simulink model "TST_SmkLim_InjMassLim"  (R2016b)
settings: Solver=FixedStepDiscrete  StartTime=0.0  StopTime=4  FixedStep=sampleTime  RelTol=1e-3
values from neighbouring files (symbols this model uses):
  testCase = 1    [initTST_SmkLim_InjMassLim_001.m]    (also in initTST_SmkLim_InjMassLim_002.m = 2)
libraries: simulink x7, UnitTest_Lib x4
settings Model: Creator=zhengjinyan  LastModifiedBy=zhengjinyan
settings DebuggingCC: SignalRangeChecking=error

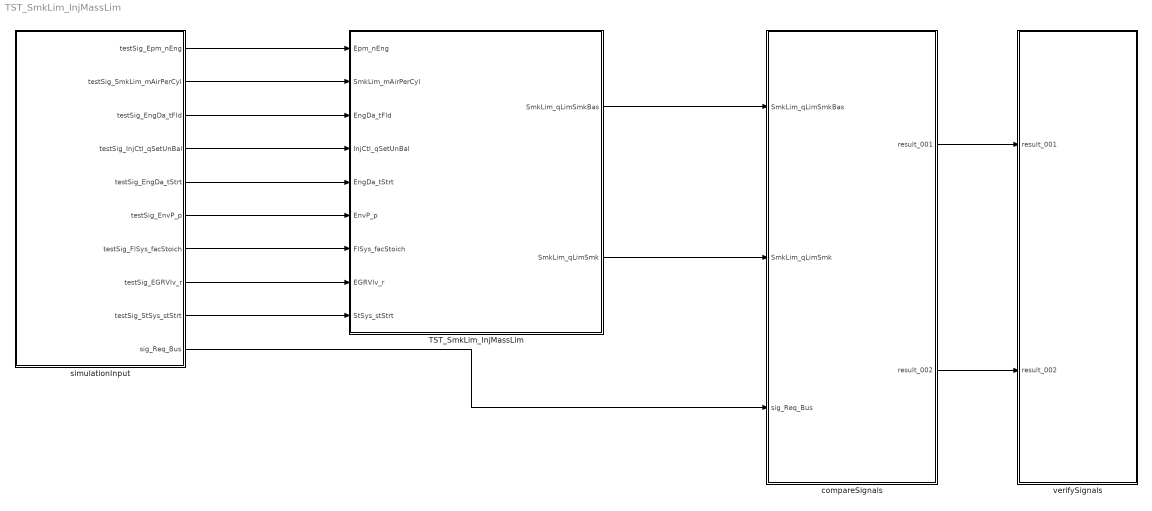
== system TST_SmkLim_InjMassLim ==
  TST_SmkLim_InjMassLim : Subsystem
  compareSignals : Subsystem
  simulationInput : Subsystem
  verifySignals : Subsystem
  wires:
  simulationInput/1(testSig_Epm_nEng) -> TST_SmkLim_InjMassLim/1(Epm_nEng)
  simulationInput/2(testSig_SmkLim_mAirPerCyl) -> TST_SmkLim_InjMassLim/2(SmkLim_mAirPerCyl)
  simulationInput/3(testSig_EngDa_tFld) -> TST_SmkLim_InjMassLim/3(EngDa_tFld)
  simulationInput/4(testSig_InjCtl_qSetUnBal) -> TST_SmkLim_InjMassLim/4(InjCtl_qSetUnBal)
  simulationInput/5(testSig_EngDa_tStrt) -> TST_SmkLim_InjMassLim/5(EngDa_tStrt)
  simulationInput/6(testSig_EnvP_p) -> TST_SmkLim_InjMassLim/6(EnvP_p)
  simulationInput/7(testSig_FlSys_facStoich) -> TST_SmkLim_InjMassLim/7(FlSys_facStoich)
  simulationInput/8(testSig_EGRVlv_r) -> TST_SmkLim_InjMassLim/8(EGRVlv_r)
  simulationInput/9(testSig_StSys_stStrt) -> TST_SmkLim_InjMassLim/9(StSys_stStrt)
  TST_SmkLim_InjMassLim/1(SmkLim_qLimSmkBas) -> compareSignals/1(SmkLim_qLimSmkBas)
  TST_SmkLim_InjMassLim/2(SmkLim_qLimSmk) -> compareSignals/2(SmkLim_qLimSmk)
  simulationInput/10(sig_Req_Bus) -> compareSignals/3(sig_Req_Bus)
  compareSignals/1(result_001) -> verifySignals/1(result_001)
  compareSignals/2(result_002) -> verifySignals/2(result_002)

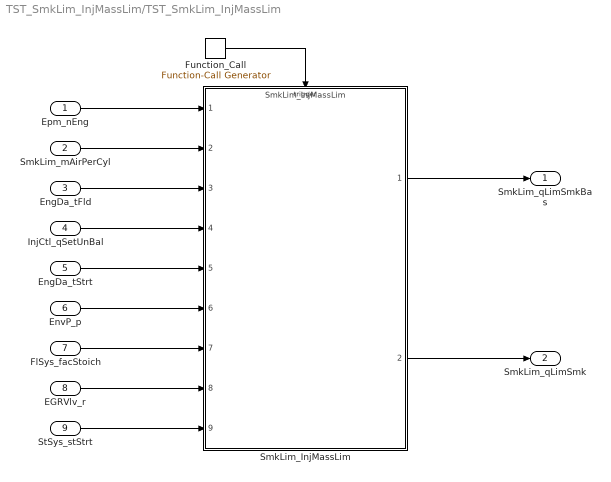
== system TST_SmkLim_InjMassLim/TST_SmkLim_InjMassLim ==
  Epm_nEng : Inport
  SmkLim_mAirPerCyl : Inport  Port=2
  EngDa_tFld : Inport  Port=3
  InjCtl_qSetUnBal : Inport  Port=4
  EngDa_tStrt : Inport  Port=5
  EnvP_p : Inport  Port=6
  FlSys_facStoich : Inport  Port=7
  EGRVlv_r : Inport  Port=8
  StSys_stStrt : Inport  Port=9
  Function_Call : simulink/Ports & Subsystems/Function-Call Generator  sample_time=sampleTime  numberOfIterations=1
  SmkLim_InjMassLim : ModelReference  ModelNameDialog=SmkLim_InjMassLim  SimulationMode=Normal  ModelReferenceVersion=1.49  TriggerPortName=function  TriggerPortTriggerType=function-call  TriggerPortStatesWhenEnabling=held
  SmkLim_qLimSmkBas : Outport
  SmkLim_qLimSmk : Outport  Port=2
  wires:
  Function_Call/1 -> SmkLim_InjMassLim/Trigger
  Epm_nEng/1 -> SmkLim_InjMassLim/1
  SmkLim_mAirPerCyl/1 -> SmkLim_InjMassLim/2
  EngDa_tFld/1 -> SmkLim_InjMassLim/3
  InjCtl_qSetUnBal/1 -> SmkLim_InjMassLim/4
  EngDa_tStrt/1 -> SmkLim_InjMassLim/5
  EnvP_p/1 -> SmkLim_InjMassLim/6
  FlSys_facStoich/1 -> SmkLim_InjMassLim/7
  EGRVlv_r/1 -> SmkLim_InjMassLim/8
  StSys_stStrt/1 -> SmkLim_InjMassLim/9
  SmkLim_InjMassLim/1 -> SmkLim_qLimSmkBas/1
  SmkLim_InjMassLim/2 -> SmkLim_qLimSmk/1

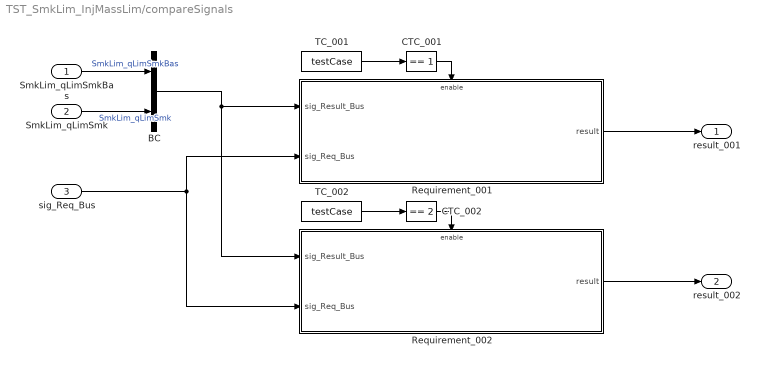
== system TST_SmkLim_InjMassLim/compareSignals ==
  SmkLim_qLimSmkBas : Inport
  SmkLim_qLimSmk : Inport  Port=2
  sig_Req_Bus : Inport  Port=3
  BC : BusCreator  Inputs=2
  CTC_001 : simulink/Logic and Bit Operations/Compare To Constant  relop===  const=1  OutDataTypeStr=boolean
  CTC_002 : simulink/Logic and Bit Operations/Compare To Constant  relop===  const=2  OutDataTypeStr=boolean
  Requirement_001 : Subsystem
  Requirement_002 : Subsystem
  TC_001 : Constant  Value=testCase
  TC_002 : Constant  Value=testCase
  result_001 : Outport
  result_002 : Outport  Port=2
  wires:
  SmkLim_qLimSmkBas/1 -> BC/1  "SmkLim_qLimSmkBas"
  SmkLim_qLimSmk/1 -> BC/2  "SmkLim_qLimSmk"
  TC_001/1 -> CTC_001/1
  CTC_001/1 -> Requirement_001/Enable
  sig_Req_Bus/1 -> Requirement_001/2(sig_Req_Bus), Requirement_002/2(sig_Req_Bus)
  BC/1 -> Requirement_001/1(sig_Result_Bus), Requirement_002/1(sig_Result_Bus)
  Requirement_001/1(result) -> result_001/1
  TC_002/1 -> CTC_002/1
  CTC_002/1 -> Requirement_002/Enable
  Requirement_002/1(result) -> result_002/1

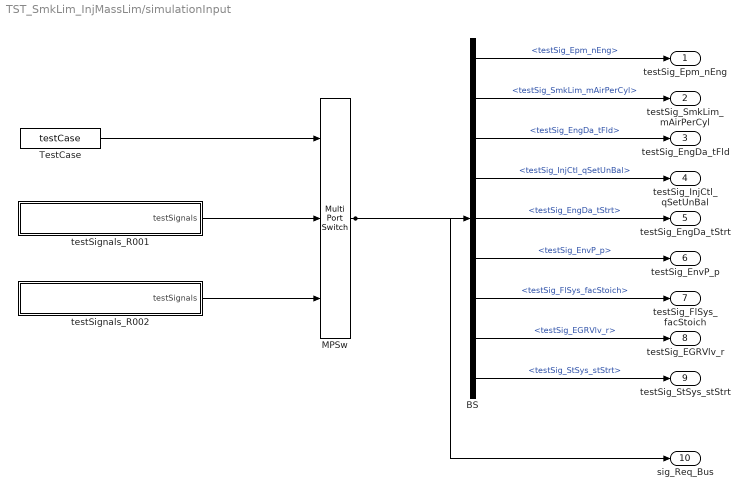
== system TST_SmkLim_InjMassLim/simulationInput ==
  BS : BusSelector  OutputSignals=testSig_Epm_nEng,testSig_SmkLim_mAirPerCyl,testSig_EngDa_tFld,testSig_InjCtl_qSetUnBal,testSig_EngDa_tStrt,testSig_EnvP_p,testSig_FlSys_facStoich,testSig_EGRVlv_r,testSig_StSys_stStrt
  MPSw : MultiPortSwitch  Inputs=2  SaturateOnIntegerOverflow=on  InputSameDT=on
  TestCase : Constant  Value=testCase
  testSignals_R001 : Subsystem
  testSignals_R002 : Subsystem
  testSig_Epm_nEng : Outport
  testSig_SmkLim_mAirPerCyl : Outport  Port=2
  testSig_EngDa_tFld : Outport  Port=3
  testSig_InjCtl_qSetUnBal : Outport  Port=4
  testSig_EngDa_tStrt : Outport  Port=5
  testSig_EnvP_p : Outport  Port=6
  testSig_FlSys_facStoich : Outport  Port=7
  testSig_EGRVlv_r : Outport  Port=8
  testSig_StSys_stStrt : Outport  Port=9
  sig_Req_Bus : Outport  Port=10
  wires:
  BS/1 -> testSig_Epm_nEng/1  "<testSig_Epm_nEng>"
  BS/2 -> testSig_SmkLim_mAirPerCyl/1  "<testSig_SmkLim_mAirPerCyl>"
  BS/3 -> testSig_EngDa_tFld/1  "<testSig_EngDa_tFld>"
  BS/4 -> testSig_InjCtl_qSetUnBal/1  "<testSig_InjCtl_qSetUnBal>"
  BS/5 -> testSig_EngDa_tStrt/1  "<testSig_EngDa_tStrt>"
  BS/6 -> testSig_EnvP_p/1  "<testSig_EnvP_p>"
  BS/7 -> testSig_FlSys_facStoich/1  "<testSig_FlSys_facStoich>"
  BS/8 -> testSig_EGRVlv_r/1  "<testSig_EGRVlv_r>"
  BS/9 -> testSig_StSys_stStrt/1  "<testSig_StSys_stStrt>"
  MPSw/1 -> BS/1, sig_Req_Bus/1
  TestCase/1 -> MPSw/1
  testSignals_R001/1(testSignals) -> MPSw/2
  testSignals_R002/1(testSignals) -> MPSw/3

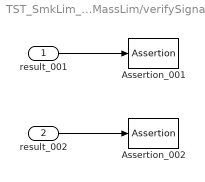
== system TST_SmkLim_InjMassLim/verifySignals ==
  result_001 : Inport
  result_002 : Inport  Port=2
  Assertion_001 : Assertion  Enabled=off
  Assertion_002 : Assertion  Enabled=off
  wires:
  result_001/1 -> Assertion_001/1
  result_002/1 -> Assertion_002/1

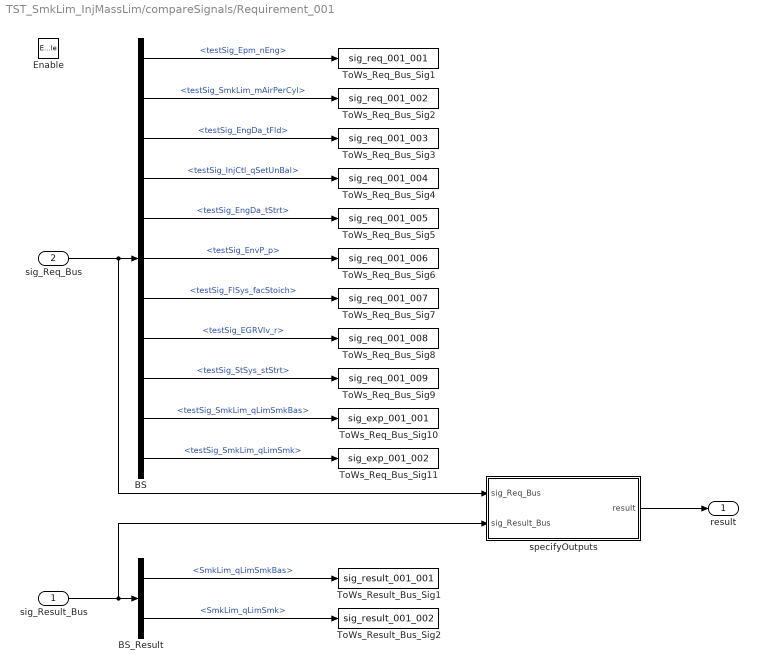
== system TST_SmkLim_InjMassLim/compareSignals/Requirement_001 ==
  sig_Result_Bus : Inport
  sig_Req_Bus : Inport  Port=2
  Enable : EnablePort
  BS : BusSelector  OutputSignals=testSig_Epm_nEng,testSig_SmkLim_mAirPerCyl,testSig_EngDa_tFld,testSig_InjCtl_qSetUnBal,testSig_EngDa_tStrt,testSig_EnvP_p,testSig_FlSys_facStoich,testSig_EGRVlv_r,testSig_StSys_stStrt,testSig_SmkLim_qLimSmkBas,testSig_SmkLim_qLimSmk
  BS_Result : BusSelector  OutputSignals=SmkLim_qLimSmkBas,SmkLim_qLimSmk
  ToWs_Req_Bus_Sig1 : ToWorkspace  VariableName=sig_req_001_001  SaveFormat=Structure With Time
  ToWs_Req_Bus_Sig10 : ToWorkspace  VariableName=sig_exp_001_001  SaveFormat=Structure With Time
  ToWs_Req_Bus_Sig11 : ToWorkspace  VariableName=sig_exp_001_002  SaveFormat=Structure With Time
  ToWs_Req_Bus_Sig2 : ToWorkspace  VariableName=sig_req_001_002  SaveFormat=Structure With Time
  ToWs_Req_Bus_Sig3 : ToWorkspace  VariableName=sig_req_001_003  SaveFormat=Structure With Time
  ToWs_Req_Bus_Sig4 : ToWorkspace  VariableName=sig_req_001_004  SaveFormat=Structure With Time
  ToWs_Req_Bus_Sig5 : ToWorkspace  VariableName=sig_req_001_005  SaveFormat=Structure With Time
  ToWs_Req_Bus_Sig6 : ToWorkspace  VariableName=sig_req_001_006  SaveFormat=Structure With Time
  ToWs_Req_Bus_Sig7 : ToWorkspace  VariableName=sig_req_001_007  SaveFormat=Structure With Time
  ToWs_Req_Bus_Sig8 : ToWorkspace  VariableName=sig_req_001_008  SaveFormat=Structure With Time
  ToWs_Req_Bus_Sig9 : ToWorkspace  VariableName=sig_req_001_009  SaveFormat=Structure With Time
  ToWs_Result_Bus_Sig1 : ToWorkspace  VariableName=sig_result_001_001  SaveFormat=Structure With Time
  ToWs_Result_Bus_Sig2 : ToWorkspace  VariableName=sig_result_001_002  SaveFormat=Structure With Time
  specifyOutputs : Subsystem
  result : Outport
  wires:
  sig_Req_Bus/1 -> BS/1, specifyOutputs/1(sig_Req_Bus)
  BS/1 -> ToWs_Req_Bus_Sig1/1  "<testSig_Epm_nEng>"
  BS/2 -> ToWs_Req_Bus_Sig2/1  "<testSig_SmkLim_mAirPerCyl>"
  BS/3 -> ToWs_Req_Bus_Sig3/1  "<testSig_EngDa_tFld>"
  BS/4 -> ToWs_Req_Bus_Sig4/1  "<testSig_InjCtl_qSetUnBal>"
  BS/5 -> ToWs_Req_Bus_Sig5/1  "<testSig_EngDa_tStrt>"
  BS/6 -> ToWs_Req_Bus_Sig6/1  "<testSig_EnvP_p>"
  BS/7 -> ToWs_Req_Bus_Sig7/1  "<testSig_FlSys_facStoich>"
  BS/8 -> ToWs_Req_Bus_Sig8/1  "<testSig_EGRVlv_r>"
  BS/9 -> ToWs_Req_Bus_Sig9/1  "<testSig_StSys_stStrt>"
  BS/10 -> ToWs_Req_Bus_Sig10/1  "<testSig_SmkLim_qLimSmkBas>"
  BS/11 -> ToWs_Req_Bus_Sig11/1  "<testSig_SmkLim_qLimSmk>"
  sig_Result_Bus/1 -> BS_Result/1, specifyOutputs/2(sig_Result_Bus)
  BS_Result/1 -> ToWs_Result_Bus_Sig1/1  "<SmkLim_qLimSmkBas>"
  BS_Result/2 -> ToWs_Result_Bus_Sig2/1  "<SmkLim_qLimSmk>"
  specifyOutputs/1(result) -> result/1

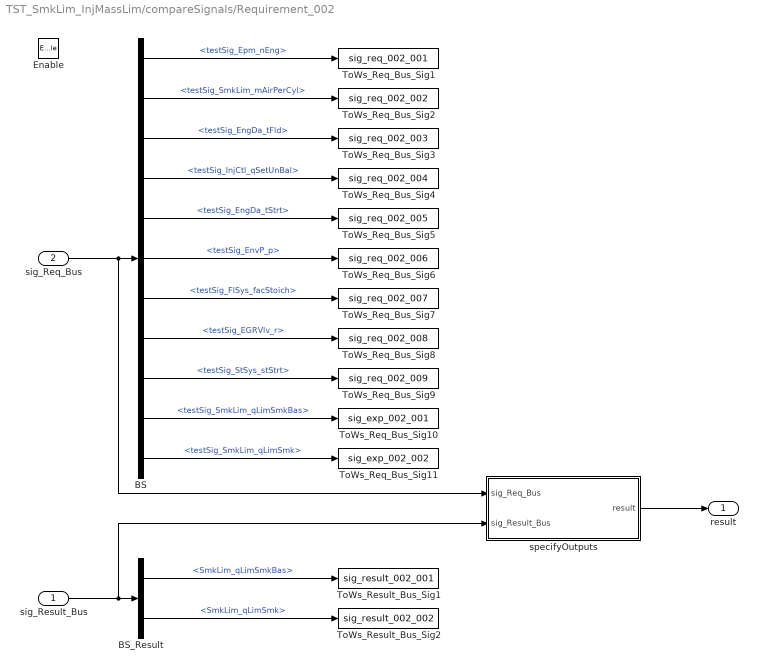
== system TST_SmkLim_InjMassLim/compareSignals/Requirement_002 ==
  sig_Result_Bus : Inport
  sig_Req_Bus : Inport  Port=2
  Enable : EnablePort
  BS : BusSelector  OutputSignals=testSig_Epm_nEng,testSig_SmkLim_mAirPerCyl,testSig_EngDa_tFld,testSig_InjCtl_qSetUnBal,testSig_EngDa_tStrt,testSig_EnvP_p,testSig_FlSys_facStoich,testSig_EGRVlv_r,testSig_StSys_stStrt,testSig_SmkLim_qLimSmkBas,testSig_SmkLim_qLimSmk
  BS_Result : BusSelector  OutputSignals=SmkLim_qLimSmkBas,SmkLim_qLimSmk
  ToWs_Req_Bus_Sig1 : ToWorkspace  VariableName=sig_req_002_001  SaveFormat=Structure With Time
  ToWs_Req_Bus_Sig10 : ToWorkspace  VariableName=sig_exp_002_001  SaveFormat=Structure With Time
  ToWs_Req_Bus_Sig11 : ToWorkspace  VariableName=sig_exp_002_002  SaveFormat=Structure With Time
  ToWs_Req_Bus_Sig2 : ToWorkspace  VariableName=sig_req_002_002  SaveFormat=Structure With Time
  ToWs_Req_Bus_Sig3 : ToWorkspace  VariableName=sig_req_002_003  SaveFormat=Structure With Time
  ToWs_Req_Bus_Sig4 : ToWorkspace  VariableName=sig_req_002_004  SaveFormat=Structure With Time
  ToWs_Req_Bus_Sig5 : ToWorkspace  VariableName=sig_req_002_005  SaveFormat=Structure With Time
  ToWs_Req_Bus_Sig6 : ToWorkspace  VariableName=sig_req_002_006  SaveFormat=Structure With Time
  ToWs_Req_Bus_Sig7 : ToWorkspace  VariableName=sig_req_002_007  SaveFormat=Structure With Time
  ToWs_Req_Bus_Sig8 : ToWorkspace  VariableName=sig_req_002_008  SaveFormat=Structure With Time
  ToWs_Req_Bus_Sig9 : ToWorkspace  VariableName=sig_req_002_009  SaveFormat=Structure With Time
  ToWs_Result_Bus_Sig1 : ToWorkspace  VariableName=sig_result_002_001  SaveFormat=Structure With Time
  ToWs_Result_Bus_Sig2 : ToWorkspace  VariableName=sig_result_002_002  SaveFormat=Structure With Time
  specifyOutputs : Subsystem
  result : Outport
  wires:
  sig_Req_Bus/1 -> BS/1, specifyOutputs/1(sig_Req_Bus)
  BS/1 -> ToWs_Req_Bus_Sig1/1  "<testSig_Epm_nEng>"
  BS/2 -> ToWs_Req_Bus_Sig2/1  "<testSig_SmkLim_mAirPerCyl>"
  BS/3 -> ToWs_Req_Bus_Sig3/1  "<testSig_EngDa_tFld>"
  BS/4 -> ToWs_Req_Bus_Sig4/1  "<testSig_InjCtl_qSetUnBal>"
  BS/5 -> ToWs_Req_Bus_Sig5/1  "<testSig_EngDa_tStrt>"
  BS/6 -> ToWs_Req_Bus_Sig6/1  "<testSig_EnvP_p>"
  BS/7 -> ToWs_Req_Bus_Sig7/1  "<testSig_FlSys_facStoich>"
  BS/8 -> ToWs_Req_Bus_Sig8/1  "<testSig_EGRVlv_r>"
  BS/9 -> ToWs_Req_Bus_Sig9/1  "<testSig_StSys_stStrt>"
  BS/10 -> ToWs_Req_Bus_Sig10/1  "<testSig_SmkLim_qLimSmkBas>"
  BS/11 -> ToWs_Req_Bus_Sig11/1  "<testSig_SmkLim_qLimSmk>"
  sig_Result_Bus/1 -> BS_Result/1, specifyOutputs/2(sig_Result_Bus)
  BS_Result/1 -> ToWs_Result_Bus_Sig1/1  "<SmkLim_qLimSmkBas>"
  BS_Result/2 -> ToWs_Result_Bus_Sig2/1  "<SmkLim_qLimSmk>"
  specifyOutputs/1(result) -> result/1

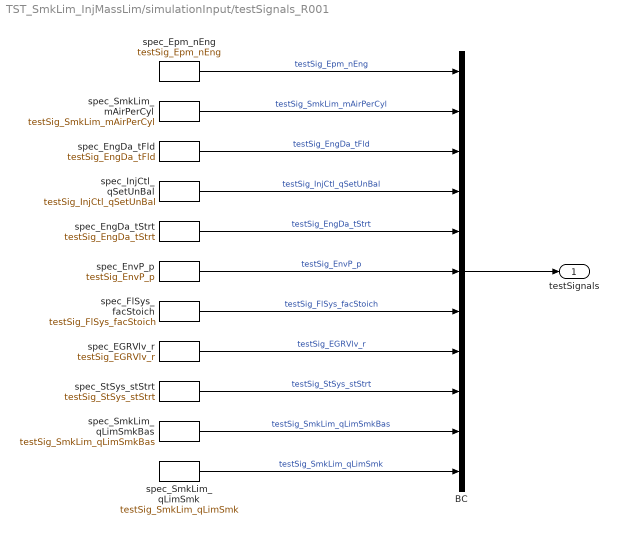
== system TST_SmkLim_InjMassLim/simulationInput/testSignals_R001 ==
  BC : BusCreator  Inputs=11
  spec_EGRVlv_r : FromWorkspace  VariableName=testSig_EGRVlv_r  Interpolate=off  OutputAfterFinalValue=Holding final value
  spec_EngDa_tFld : FromWorkspace  VariableName=testSig_EngDa_tFld  Interpolate=off  OutputAfterFinalValue=Holding final value
  spec_EngDa_tStrt : FromWorkspace  VariableName=testSig_EngDa_tStrt  Interpolate=off  OutputAfterFinalValue=Holding final value
  spec_EnvP_p : FromWorkspace  VariableName=testSig_EnvP_p  Interpolate=off  OutputAfterFinalValue=Holding final value
  spec_Epm_nEng : FromWorkspace  VariableName=testSig_Epm_nEng  Interpolate=off  OutputAfterFinalValue=Holding final value
  spec_FlSys_facStoich : FromWorkspace  VariableName=testSig_FlSys_facStoich  Interpolate=off  OutputAfterFinalValue=Holding final value
  spec_InjCtl_qSetUnBal : FromWorkspace  VariableName=testSig_InjCtl_qSetUnBal  Interpolate=off  OutputAfterFinalValue=Holding final value
  spec_SmkLim_mAirPerCyl : FromWorkspace  VariableName=testSig_SmkLim_mAirPerCyl  Interpolate=off  OutputAfterFinalValue=Holding final value
  spec_SmkLim_qLimSmk : FromWorkspace  VariableName=testSig_SmkLim_qLimSmk  Interpolate=off  OutputAfterFinalValue=Holding final value
  spec_SmkLim_qLimSmkBas : FromWorkspace  VariableName=testSig_SmkLim_qLimSmkBas  Interpolate=off  OutputAfterFinalValue=Holding final value
  spec_StSys_stStrt : FromWorkspace  VariableName=testSig_StSys_stStrt  Interpolate=off  OutputAfterFinalValue=Holding final value
  testSignals : Outport
  wires:
  BC/1 -> testSignals/1
  spec_Epm_nEng/1 -> BC/1  "testSig_Epm_nEng"
  spec_SmkLim_mAirPerCyl/1 -> BC/2  "testSig_SmkLim_mAirPerCyl"
  spec_EngDa_tFld/1 -> BC/3  "testSig_EngDa_tFld"
  spec_InjCtl_qSetUnBal/1 -> BC/4  "testSig_InjCtl_qSetUnBal"
  spec_EngDa_tStrt/1 -> BC/5  "testSig_EngDa_tStrt"
  spec_EnvP_p/1 -> BC/6  "testSig_EnvP_p"
  spec_FlSys_facStoich/1 -> BC/7  "testSig_FlSys_facStoich"
  spec_EGRVlv_r/1 -> BC/8  "testSig_EGRVlv_r"
  spec_StSys_stStrt/1 -> BC/9  "testSig_StSys_stStrt"
  spec_SmkLim_qLimSmkBas/1 -> BC/10  "testSig_SmkLim_qLimSmkBas"
  spec_SmkLim_qLimSmk/1 -> BC/11  "testSig_SmkLim_qLimSmk"

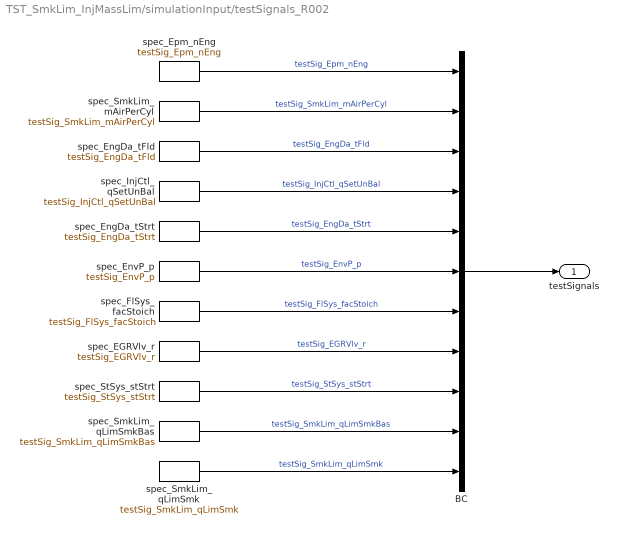
== system TST_SmkLim_InjMassLim/simulationInput/testSignals_R002 ==
  BC : BusCreator  Inputs=11
  spec_EGRVlv_r : FromWorkspace  VariableName=testSig_EGRVlv_r  Interpolate=off  OutputAfterFinalValue=Holding final value
  spec_EngDa_tFld : FromWorkspace  VariableName=testSig_EngDa_tFld  Interpolate=off  OutputAfterFinalValue=Holding final value
  spec_EngDa_tStrt : FromWorkspace  VariableName=testSig_EngDa_tStrt  Interpolate=off  OutputAfterFinalValue=Holding final value
  spec_EnvP_p : FromWorkspace  VariableName=testSig_EnvP_p  Interpolate=off  OutputAfterFinalValue=Holding final value
  spec_Epm_nEng : FromWorkspace  VariableName=testSig_Epm_nEng  Interpolate=off  OutputAfterFinalValue=Holding final value
  spec_FlSys_facStoich : FromWorkspace  VariableName=testSig_FlSys_facStoich  Interpolate=off  OutputAfterFinalValue=Holding final value
  spec_InjCtl_qSetUnBal : FromWorkspace  VariableName=testSig_InjCtl_qSetUnBal  Interpolate=off  OutputAfterFinalValue=Holding final value
  spec_SmkLim_mAirPerCyl : FromWorkspace  VariableName=testSig_SmkLim_mAirPerCyl  Interpolate=off  OutputAfterFinalValue=Holding final value
  spec_SmkLim_qLimSmk : FromWorkspace  VariableName=testSig_SmkLim_qLimSmk  Interpolate=off  OutputAfterFinalValue=Holding final value
  spec_SmkLim_qLimSmkBas : FromWorkspace  VariableName=testSig_SmkLim_qLimSmkBas  Interpolate=off  OutputAfterFinalValue=Holding final value
  spec_StSys_stStrt : FromWorkspace  VariableName=testSig_StSys_stStrt  Interpolate=off  OutputAfterFinalValue=Holding final value
  testSignals : Outport
  wires:
  BC/1 -> testSignals/1
  spec_Epm_nEng/1 -> BC/1  "testSig_Epm_nEng"
  spec_SmkLim_mAirPerCyl/1 -> BC/2  "testSig_SmkLim_mAirPerCyl"
  spec_EngDa_tFld/1 -> BC/3  "testSig_EngDa_tFld"
  spec_InjCtl_qSetUnBal/1 -> BC/4  "testSig_InjCtl_qSetUnBal"
  spec_EngDa_tStrt/1 -> BC/5  "testSig_EngDa_tStrt"
  spec_EnvP_p/1 -> BC/6  "testSig_EnvP_p"
  spec_FlSys_facStoich/1 -> BC/7  "testSig_FlSys_facStoich"
  spec_EGRVlv_r/1 -> BC/8  "testSig_EGRVlv_r"
  spec_StSys_stStrt/1 -> BC/9  "testSig_StSys_stStrt"
  spec_SmkLim_qLimSmkBas/1 -> BC/10  "testSig_SmkLim_qLimSmkBas"
  spec_SmkLim_qLimSmk/1 -> BC/11  "testSig_SmkLim_qLimSmk"

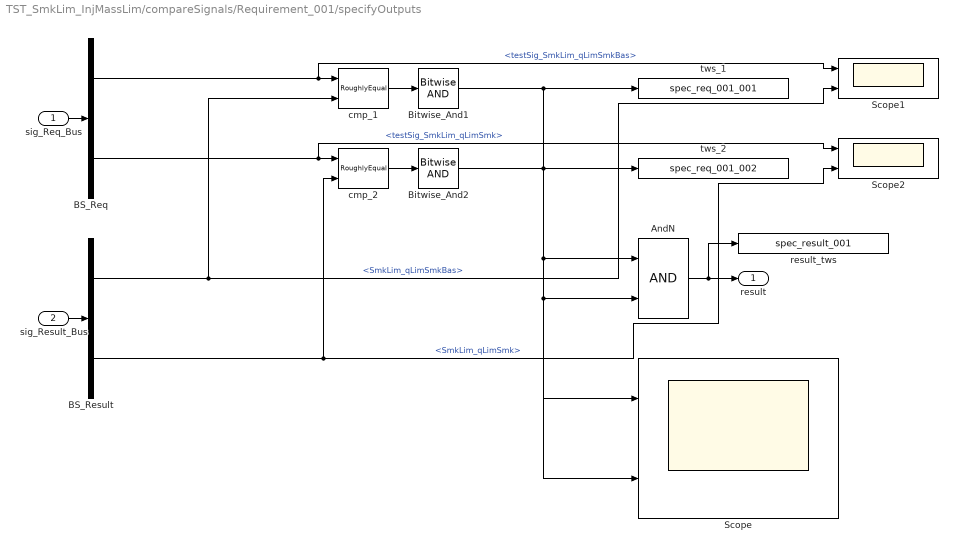
== system TST_SmkLim_InjMassLim/compareSignals/Requirement_001/specifyOutputs ==
  sig_Req_Bus : Inport
  sig_Result_Bus : Inport  Port=2
  AndN : Logic
  BS_Req : BusSelector  OutputSignals=testSig_SmkLim_qLimSmkBas,testSig_SmkLim_qLimSmk
  BS_Result : BusSelector  OutputSignals=SmkLim_qLimSmkBas,SmkLim_qLimSmk
  Bitwise_And1 : simulink/Logic and Bit Operations/Bitwise Operator  logicop=AND  UseBitMask=off  BitMask=bin2dec('11011001')  BitMaskRealWorld=Stored Integer
  Bitwise_And2 : simulink/Logic and Bit Operations/Bitwise Operator  logicop=AND  UseBitMask=off  BitMask=bin2dec('11011001')  BitMaskRealWorld=Stored Integer
  Scope : Scope  NumInputPorts=2
  Scope1 : Scope  NumInputPorts=2
  Scope2 : Scope  NumInputPorts=2
  cmp_1 : UnitTest_Lib/RoughlyEqual  slope=1
  cmp_2 : UnitTest_Lib/RoughlyEqual  slope=1
  result_tws : ToWorkspace  VariableName=spec_result_001
  tws_1 : ToWorkspace  VariableName=spec_req_001_001
  tws_2 : ToWorkspace  VariableName=spec_req_001_002
  result : Outport
  wires:
  sig_Req_Bus/1 -> BS_Req/1
  sig_Result_Bus/1 -> BS_Result/1
  AndN/1 -> result/1, result_tws/1
  BS_Req/1 -> cmp_1/1, Scope1/1  "<testSig_SmkLim_qLimSmkBas>"
  BS_Result/1 -> cmp_1/2, Scope1/2  "<SmkLim_qLimSmkBas>"
  cmp_1/1 -> Bitwise_And1/1
  Bitwise_And1/1 -> AndN/1, Scope/1, tws_1/1
  BS_Req/2 -> cmp_2/1, Scope2/1  "<testSig_SmkLim_qLimSmk>"
  BS_Result/2 -> cmp_2/2, Scope2/2  "<SmkLim_qLimSmk>"
  cmp_2/1 -> Bitwise_And2/1
  Bitwise_And2/1 -> AndN/2, Scope/2, tws_2/1

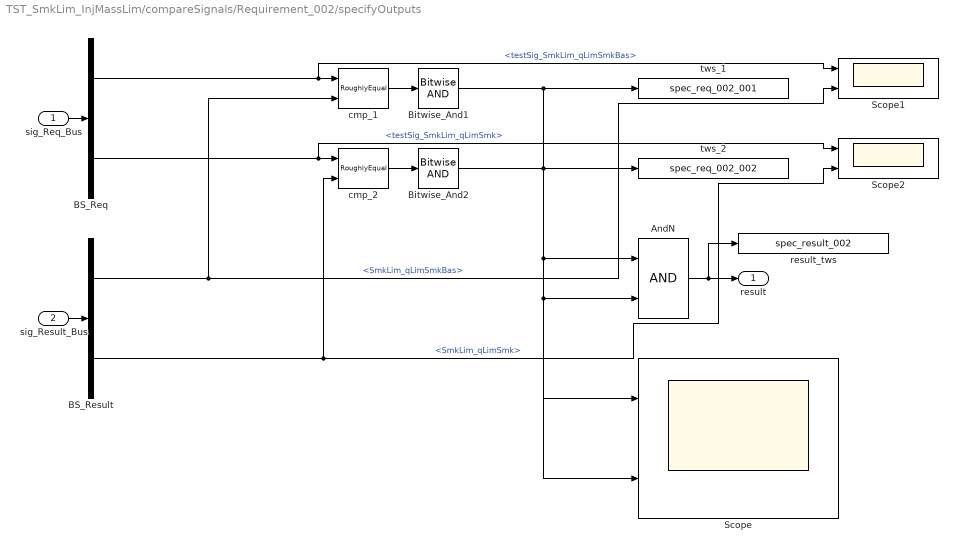
== system TST_SmkLim_InjMassLim/compareSignals/Requirement_002/specifyOutputs ==
  sig_Req_Bus : Inport
  sig_Result_Bus : Inport  Port=2
  AndN : Logic
  BS_Req : BusSelector  OutputSignals=testSig_SmkLim_qLimSmkBas,testSig_SmkLim_qLimSmk
  BS_Result : BusSelector  OutputSignals=SmkLim_qLimSmkBas,SmkLim_qLimSmk
  Bitwise_And1 : simulink/Logic and Bit Operations/Bitwise Operator  logicop=AND  UseBitMask=off  BitMask=bin2dec('11011001')  BitMaskRealWorld=Stored Integer
  Bitwise_And2 : simulink/Logic and Bit Operations/Bitwise Operator  logicop=AND  UseBitMask=off  BitMask=bin2dec('11011001')  BitMaskRealWorld=Stored Integer
  Scope : Scope  NumInputPorts=2
  Scope1 : Scope  NumInputPorts=2
  Scope2 : Scope  NumInputPorts=2
  cmp_1 : UnitTest_Lib/RoughlyEqual  slope=1
  cmp_2 : UnitTest_Lib/RoughlyEqual  slope=1
  result_tws : ToWorkspace  VariableName=spec_result_002
  tws_1 : ToWorkspace  VariableName=spec_req_002_001
  tws_2 : ToWorkspace  VariableName=spec_req_002_002
  result : Outport
  wires:
  sig_Req_Bus/1 -> BS_Req/1
  sig_Result_Bus/1 -> BS_Result/1
  AndN/1 -> result/1, result_tws/1
  BS_Req/1 -> cmp_1/1, Scope1/1  "<testSig_SmkLim_qLimSmkBas>"
  BS_Result/1 -> cmp_1/2, Scope1/2  "<SmkLim_qLimSmkBas>"
  cmp_1/1 -> Bitwise_And1/1
  Bitwise_And1/1 -> AndN/1, Scope/1, tws_1/1
  BS_Req/2 -> cmp_2/1, Scope2/1  "<testSig_SmkLim_qLimSmk>"
  BS_Result/2 -> cmp_2/2, Scope2/2  "<SmkLim_qLimSmk>"
  cmp_2/1 -> Bitwise_And2/1
  Bitwise_And2/1 -> AndN/2, Scope/2, tws_2/1
